simulink model "simulink_recursive_solve"  (R2025b)
settings: Solver=VariableStepAuto  StartTime=0.0  StopTime=10.0  RelTol=1e-3
values from neighbouring files (symbols this model uses):
  A_c = L_SIDE^2 - L*t*N    [constants_part2.m]    (also in constants_part2_3.m; perf.m)
  c_p = 1006    [constants_part1.m]    (also in constants_part2.m = 1007; constants_part2_3.m = 1007; constants_part3.m = 1007)
  D_h = (2*L*s)/(L+s)    [constants_part2.m]    (also in constants_part2_3.m; perf.m)
  k = 178    [constants_part1.m]
  L = 0.025    [constants.m]
  L_DUCT = 0.15    [constants.m]
  L_SIDE = 0.15    [constants.m]
  N = 24*4    (= 96)    [constants.m]
  nu = 1.655e-5    (= 1.655e-05)    [constants_part2.m]    (also in constants_part3.m; iterative_solver.m = 0.0001655; iterative_solver2.m = 0.0001655; part2.m = 0.0001655)
  Pr = 0.7268    [constants_part2.m]    (also in constants_part3.m; iterative_solver.m; iterative_solver2.m; part2.m)
  R_cond = t_DUCT/(k * A_c_wall)    [iterative_solver.m]    (also in iterative_solver2.m; part2.m; part2_old.m = t_DUCT/(k_duct * A_c_walls); qdot.m = t_DUCT/(k_duct * A_c_walls))
  R_paste = 1/(h_c * A_c_CPUs)    [iterative_solver.m]    (also in iterative_solver2.m; part2.m; part2_old.m; qdot.m)
  rho = 1.14    [constants_part1.m]    (also in constants_part2.m = 1.145; constants_part3.m = 1.145; iterative_solver.m = 1.145; iterative_solver2.m = 1145)
  T_bulk = (T_me + T_mi)/2 - 273.15    [iterative_solver.m]    (also in iterative_solver2.m; part2.m; part2_old.m = (T_me + T_mi)/2; qdot.m = (T_me + T_mi)/2)
  T_me = Q_dot_tot/(m_dot_air * c_p) +T_mi    [tinf.m]
  T_mi = 20    [constants_part2.m]    (also in constants_part2_3.m; constants_part3.m)
  w = L_DUCT    (= 0.15)    [constants.m]
settings Model: Creator=simon  LastModifiedBy=simon

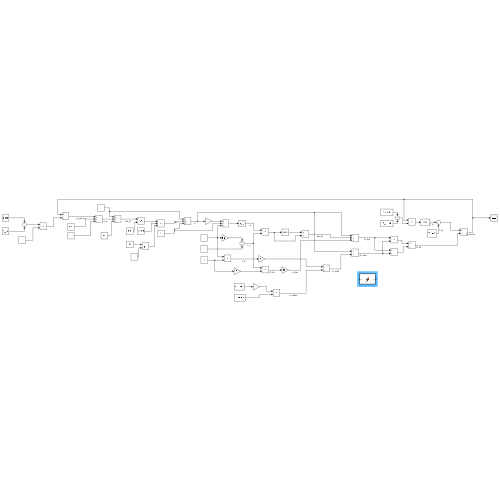
[thumbnail: Simulink's stored preview of the top-level diagram]
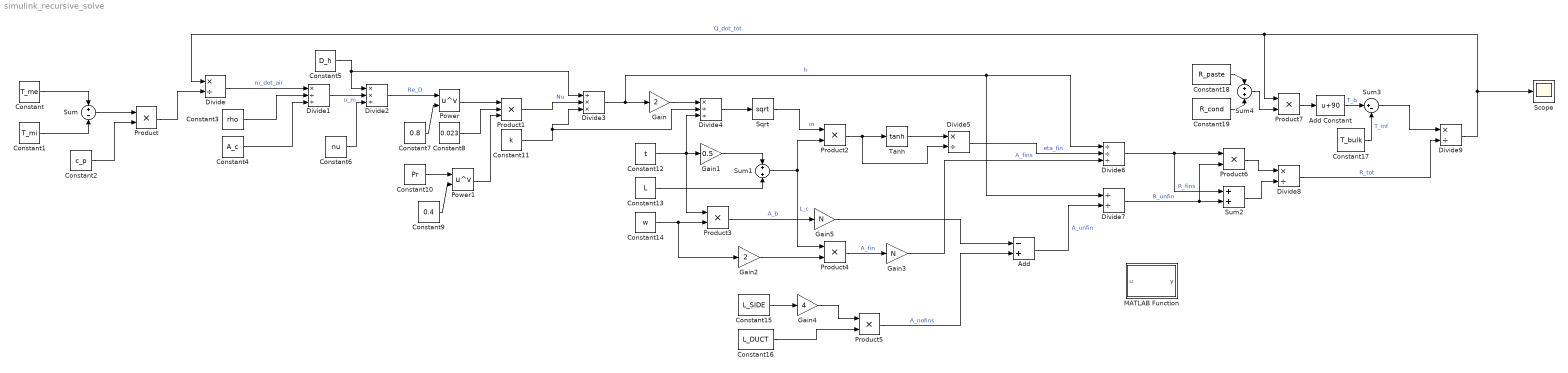
== system simulink_recursive_solve ==
  Add : Sum  Inputs=-+
  Add Constant : Bias  Bias=90  SaturateOnIntegerOverflow=off
  Constant : Constant  Value=T_me
  Constant1 : Constant  Value=T_mi
  Constant10 : Constant  Value=Pr
  Constant11 : Constant  Value=k
  Constant12 : Constant  Value=t
  Constant13 : Constant  Value=L
  Constant14 : Constant  Value=w
  Constant15 : Constant  Value=L_SIDE
  Constant16 : Constant  Value=L_DUCT
  Constant17 : Constant  Value=T_bulk
  Constant18 : Constant  Value=R_paste
  Constant19 : Constant  Value=R_cond
  Constant2 : Constant  Value=c_p
  Constant3 : Constant  Value=rho
  Constant4 : Constant  Value=A_c
  Constant5 : Constant  Value=D_h
  Constant6 : Constant  Value=nu
  Constant7 : Constant  Value=0.8
  Constant8 : Constant  Value=0.023
  Constant9 : Constant  Value=0.4
  Divide{,5,8..9} (4 alike) : Product  Inputs=*/
  Divide1 : Product  Inputs=*//
  Divide2 : Product  Inputs=**/
  Divide3 : Product  Inputs=/**
  Divide4 : Product  Inputs=*//
  Divide6 : Product  Inputs=///
  Divide7 : Product  Inputs=//
  Gain : Gain  Gain=2
  Gain1 : Gain  Gain=0.5
  Gain2 : Gain  Gain=2
  Gain3 : Gain  Gain=N
  Gain4 : Gain  Gain=4
  Gain5 : Gain  Gain=N
  MATLAB Function : MATLAB Function  TreatAsAtomicUnit=on
  Power : Math  Operator=pow
  Power1 : Math  Operator=pow
  Product{,2..7} (7 alike) : Product
  Product1 : Product  Inputs=3
  Scope : Scope
  Sqrt : Sqrt
  Sum : Sum  Inputs=+-
  Sum1 : Sum
  Sum2 : Sum
  Sum3 : Sum  Inputs=|+-
  Sum4 : Sum
  Tanh : Trigonometry  Operator=tanh
  wires:
  Constant/1 -> Sum/1
  Constant1/1 -> Sum/2
  Sum/1 -> Product/1
  Constant2/1 -> Product/2
  Product/1 -> Divide/2
  Divide/1 -> Divide1/1  "m_dot_air"
  Constant3/1 -> Divide1/2
  Constant4/1 -> Divide1/3
  Divide1/1 -> Divide2/2  "u_m"
  Constant5/1 -> Divide3/1, Divide2/1
  Constant6/1 -> Divide2/3
  Divide2/1 -> Power/1  "Re_D"
  Constant7/1 -> Power/2
  Power/1 -> Product1/1
  Constant8/1 -> Product1/2
  Constant9/1 -> Power1/2
  Power1/1 -> Product1/3
  Constant10/1 -> Power1/1
  Product1/1 -> Divide3/2  "Nu"
  Constant11/1 -> Divide4/2, Divide3/3
  Divide3/1 -> Divide7/1, Divide6/1, Gain/1  "h"
  Gain/1 -> Divide4/1
  Constant12/1 -> Product3/1, Gain1/1, Divide4/3
  Divide4/1 -> Sqrt/1
  Sqrt/1 -> Product2/1  "m"
  Gain1/1 -> Sum1/1
  Constant13/1 -> Sum1/2
  Sum1/1 -> Product4/1, Product2/2  "L_c"
  Product2/1 -> Divide5/2, Tanh/1
  Tanh/1 -> Divide5/1
  Divide5/1 -> Divide6/2  "eta_fin"
  Constant14/1 -> Gain2/1, Product3/2
  Product3/1 -> Gain5/1  "A_b"
  Gain2/1 -> Product4/2
  Product4/1 -> Gain3/1  "A_fin"
  Gain3/1 -> Divide6/3  "A_fins"
  Constant15/1 -> Gain4/1
  Gain4/1 -> Product5/1
  Constant16/1 -> Product5/2
  Product5/1 -> Add/2  "A_nofins"
  Gain5/1 -> Add/1
  Add/1 -> Divide7/2  "A_unfin"
  Divide6/1 -> Product6/1, Sum2/1  "R_fins"
  Divide7/1 -> Product6/2, Sum2/2  "R_unfin"
  Product6/1 -> Divide8/1
  Sum2/1 -> Divide8/2
  Sum3/1 -> Divide9/1
  Product7/1 -> Add Constant/1
  Constant17/1 -> Sum3/2  "T_inf"
  Divide8/1 -> Divide9/2  "R_tot"
  Divide9/1 -> Scope/1, Product7/1, Divide/1  "Q_dot_tot"
  Constant18/1 -> Sum4/1
  Constant19/1 -> Sum4/2
  Sum4/1 -> Product7/2
  Add Constant/1 -> Sum3/1  "T_b"

== matlab function simulink_recursive_solve/MATLAB Function ==
  data: u input; y output
function y = fcn(u)

y = u;
